simulink model "flight"  (R2020b)
settings: Solver=ode45  StartTime=0.0  StopTime=350  RelTol=1e-3
values from neighbouring files (symbols this model uses):
  g = 1.4    [CFD_in_CD_nozzle.m]    (also in nozzle_cfd.m; supersonic_flow_over_a_flat_plate.m)
undefined symbols (not defined in the file or in its folder): gam_0, gam_in, h_0, m_dot, m_nofuel, R_e, t_turn, v_0, x_0
libraries: simulink x1, pid_lib x1
settings Model: Creator=manavbathija  LastModifiedBy=manavbathija

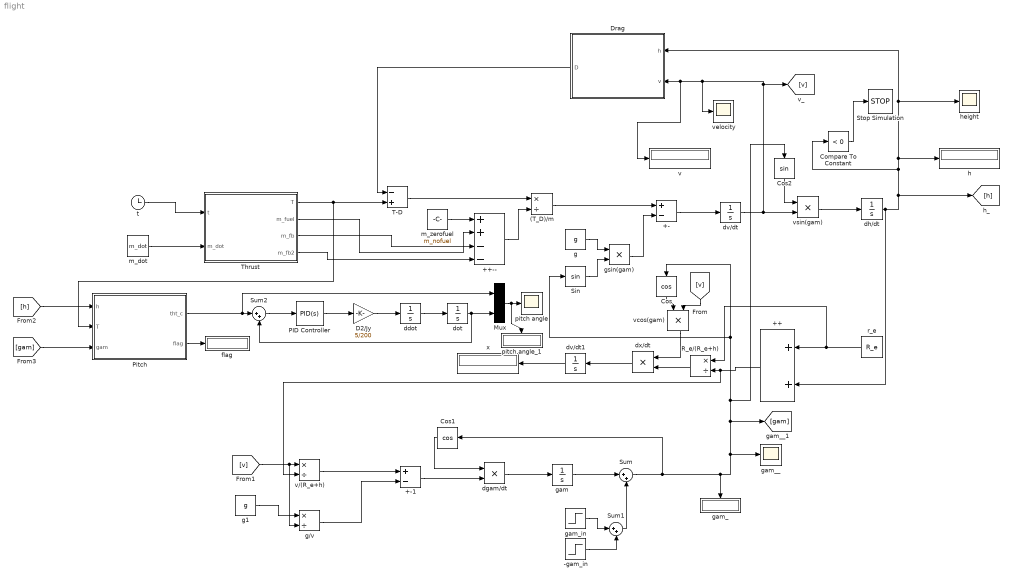
== system flight ==
  (T_D)/m : Product  Inputs=*/
  ++ : Sum
  ++-- : Sum  Inputs=++--
  +- : Sum  Inputs=+-
  +-1 : Sum  Inputs=+-
  -gam_in : Step  Time=t_turn  Before=-gam_in  After=-gam_in  SampleTime=0
  Compare To Constant : simulink/Logic and Bit Operations/Compare To Constant  relop=<  const=0  OutDataTypeStr=boolean
  Cos : Trigonometry  Operator=cos
  Cos1 : Trigonometry  Operator=cos
  Cos2 : Trigonometry
  D2/Jy : Gain  Gain=5/200
  Drag : MATLAB Function  TreatAsAtomicUnit=on
  Mux : Mux  Inputs=2
  PID Controller : pid_lib/PID Controller  Controller=PID  Form=Parallel  TimeDomain=Continuous-time  UseExternalTs=off  SampleTime=-1  IntegratorMethod=Forward Euler  FilterMethod=Forward Euler  ControllerParametersSource=internal  P=0  I=0  D=200/5  UseFilter=on  N=100  TunerSelectOption=Transfer Function Based (PID Tuner App)  InitialConditionSource=internal  InitialConditionForIntegrator=0  InitialConditionForFilter=0  DifferentiatorICPrevScaledInput=0  ExternalReset=none  TrackingMode=off  Kt=1  LimitOutput=off  SatLimitsSource=internal  UpperSaturationLimit=inf  LowerSaturationLimit=-inf  LinearizeAsGain=on  AntiWindupMode=none  Kb=1  POutMin=[]  POutMax=[]  IOutMin=[]  IOutMax=[]  DOutMin=[]  DOutMax=[]  NOutMin=[]  NOutMax=[]  SumOutMin=[]  SumOutMax=[]  SaturationOutMin=[]  SaturationOutMax=[]  PParamMin=[]  PParamMax=[]  IParamMin=[]  IParamMax=[]  DParamMin=[]  DParamMax=[]  NParamMin=[]  NParamMax=[]  KbParamMin=[]  KbParamMax=[]  KtParamMin=[]  KtParamMax=[]  KbOutMin=[]  KbOutMax=[]  KtOutMin=[]  KtOutMax=[]  IntegratorOutMin=[]  IntegratorOutMax=[]  FilterOutMin=[]  FilterOutMax=[]  SumI1OutMin=[]  SumI1OutMax=[]  SumI2OutMin=[]  SumI2OutMax=[]  SumI3OutMin=[]  SumI3OutMax=[]  SumI4OutMin=[]  SumI4OutMax=[]  SumDOutMin=[]  SumDOutMax=[]  DifferentiatorOutMin=[]  DifferentiatorOutMax=[]  FilterDiffOutCoefMin=[]  FilterDiffOutCoefMax=[]  ReciprocalOutMin=[]  ReciprocalOutMax=[]  SumDenOutMin=[]  SumDenOutMax=[]  SumNumOutMin=[]  SumNumOutMax=[]  DivideOutMin=[]  DivideOutMax=[]  UdiffTsProdOutMin=[]  UdiffTsProdOutMax=[]  NTsProdOutMin=[]  NTsProdOutMax=[]  UintegralTsProdOutMin=[]  UintegralTsProdOutMax=[]  UngainTsProdOutMin=[]  UngainTsProdOutMax=[]  IntegratorContinuousStateAttributes=''  IntegratorStateMustResolveToSignalObject=off  IntegratorRTWStateStorageClass=Auto  FilterContinuousStateAttributes=''  FilterStateMustResolveToSignalObject=off  FilterRTWStateStorageClass=Auto  ParallelPVariant=InternalParameters  IdealPVariant=Disabled  IVariant=InternalParameters  DVariant=InternalParameters  IntegratorVariant=Continuous  SatVariant=Disabled  AWVariant=Passthrough  PCopyVariant=Disabled  TRVariant=Disabled  FdbkBlocksVariant=Forward  IdealPFdbkVariant=Disabled  SatFdbkVariant=Disabled  DerivativeFilterVariant=ContFilter  NVariant=InternalParameters  NCopyVariant=Disabled  FilterICVariant=InternalICsFilter  IntegratorICVariant=InternalICs  ExternalResetVariant=Disabled  TRSumVariant=Passthrough  SumFdbkVariant=Disabled  SumVariant=Sum_PID  TsampFilterVariant=InternalTs  TsampNgainVariant=Passthrough  TsampIntegralVariant=Passthrough  ExternalSaturationOutDataTypeStr=Inherit: Same as second input
  Pitch : MATLAB Function  TreatAsAtomicUnit=on
  R_e/(R_e+h) : Product  Inputs=*/
  Sin : Trigonometry
  Stop Simulation : Stop
  Sum : Sum  Inputs=|++
  Sum1 : Sum  Inputs=|++
  Sum2 : Sum  Inputs=|++
  T-D : Sum  Inputs=-+
  Thrust : MATLAB Function  TreatAsAtomicUnit=on
  ddot : Integrator  InitialCondition=gam_0
  dgam/dt : Product
  dh/dt : Integrator  InitialCondition=h_0
  dot : Integrator
  dv/dt : Integrator  InitialCondition=v_0
  dv/dt1 : Integrator  InitialCondition=x_0
  dx/dt : Product
  flag : Display
  g : Constant  Value=g
  g/v : Product  Inputs=*/
  g1 : Constant  Value=g
  gam : Integrator  InitialCondition=gam_0
  gam_ : Display
  gam__ : Scope
  gam_in : Step  Time=t_turn  Before=gam_in  After=0  SampleTime=0
  gsin(gam) : Product
  h : Display
  height : Scope
  m_dot : Constant  Value=m_dot
  m_zerofuel : Constant  Value=m_nofuel
  pitch angle : Scope
  pitch angle_1 : Display
  r_e : Constant  Value=R_e
  t : Clock
  v : Display
  v/(R_e+h) : Product  Inputs=*/
  vcos(gam) : Product
  velocity : Scope
  vsin(gam) : Product
  x : Display
  wires:
  t/1 -> Thrust/1(t)
  m_dot/1 -> Thrust/2(m_dot)
  Thrust/1(T) -> Pitch/2(T), T-D/2
  m_zerofuel/1 -> ++--/1
  Thrust/2(m_fuel) -> ++--/2
  Thrust/3(m_fb) -> ++--/3
  Thrust/4(m_fb2) -> ++--/4
  T-D/1 -> (T_D)/m/1
  ++--/1 -> (T_D)/m/2
  (T_D)/m/1 -> +-/1
  g/1 -> gsin(gam)/1
  Sin/1 -> gsin(gam)/2
  gsin(gam)/1 -> +-/2
  +-/1 -> dv/dt/1
  dv/dt/1 -> velocity/1, v/1, Drag/2(v), [v], vsin(gam)/2
  vsin(gam)/1 -> dh/dt/1
  dh/dt/1 -> ++/2, h/1, height/1, Drag/1(h), Compare To Constant/1, [h]
  Compare To Constant/1 -> Stop Simulation/1
  Drag/1(D) -> T-D/1
  r_e/1 -> R_e/(R_e+h)/1, ++/1
  ++/1 -> v/(R_e+h)/2, R_e/(R_e+h)/2
  R_e/(R_e+h)/1 -> dx/dt/2
  Cos/1 -> vcos(gam)/1
  [v] -> vcos(gam)/2
  vcos(gam)/1 -> dx/dt/1
  dx/dt/1 -> dv/dt1/1
  dv/dt1/1 -> x/1
  [v] -> g/v/2, v/(R_e+h)/1
  v/(R_e+h)/1 -> +-1/1
  g1/1 -> g/v/1
  g/v/1 -> +-1/2
  +-1/1 -> dgam/dt/2
  Cos1/1 -> dgam/dt/1
  dgam/dt/1 -> gam/1
  gam/1 -> Sum/1
  Sum/1 -> Cos1/1, gam_/1, [gam], Cos2/1, Sin/1, Cos/1, gam__/1
  gam_in/1 -> Sum1/1
  -gam_in/1 -> Sum1/2
  Sum1/1 -> Sum/2
  [h] -> Pitch/1(h)
  [gam] -> Pitch/3(gam)
  Pitch/2(flag) -> flag/1
  Pitch/1(tht_c) -> Mux/1, Sum2/1
  Sum2/1 -> PID Controller/1
  PID Controller/1 -> D2/Jy/1
  D2/Jy/1 -> ddot/1
  ddot/1 -> dot/1
  dot/1 -> Sum2/2, Mux/2
  Mux/1 -> pitch angle_1/1, pitch angle/1
  Cos2/1 -> vsin(gam)/1

== matlab function flight/Pitch ==
  settings: updateMethod=DISCRETE
  data: h input; T input; gam input; tht_c output; flag output
function [tht_c,flag]=fcn(h,T ,gam)

persistent f
if isempty(f)
    f=0;
end

if T<=0
    t_c=gam+pi;
    if t_c>pi
        t_c=pi;
    end
    f=1;
elseif T<=0 && h<1000
    t_c=pi/2;
else
    t_c=gam;
end
flag=f;
tht_c=t_c;

== matlab function flight/Thrust ==
  settings: updateMethod=DISCRETE
  data: t input; T output; m_fuel output; m_fb output; m_fb2 output; m_dot input
function [T,m_fuel,m_fb,m_fb2] = fcn(t,m_dot)

persistent mfb
persistent mfb2

if isempty(mfb)
    mfb=0;
end
if isempty(mfb2)
    mfb2=0;
end
mfuel=21491.26;

if mfb<=0.65*mfuel
    thr=346961.2;
    mfb=t*m_dot;
else
    thr=0;
end

if 125<t && t<295
    thr=-110000;
    mfb2=(t-125)*(m_dot/3);
end
T=thr;
m_fb=mfb;
m_fb2=mfb2;
m_fuel=mfuel;

== matlab function flight/Drag ==
  data: h input; D output; v input
function D = fcn(h,v)

Cd=0.075;
Di=1.5;
A=pi*Di^2/4;

%ISA Model
if h<11000
    T=15.04-0.00649*h;
    p=101.29*((T+273.1)/288.08)^5.258;
elseif 11000<h && h<25000
    T=-56.46;
    p=22.65*exp(1.73-0.000157*h);
else
    T=-131.21+0.00299*h;
    p=2.488*((T+273.1)/216.6)^-11.388;
end
rho=p/(0.2869*(T+273.1));

Drag=0.5*rho*v^2*A*Cd;
D=Drag;
